simulink library "nonlinlib_config"  (R2013a)
settings: Solver=VariableStepDiscrete  StartTime=0.0  StopTime=10.0  RelTol=1e-3
undefined symbols (not defined in the file or in its folder): Nonlinearity, Tanh
libraries: nonlinlib x1
settings Model: Creator=bbhattac  LastModifiedBy=bbhattac

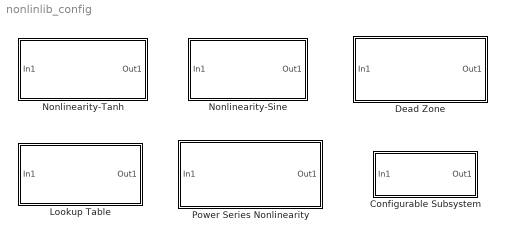
== system nonlinlib_config ==
  Configurable Subsystem : Subsystem  BlockChoice=Nonlinearity-Tanh
      settings: TemplateBlock=self  MemberBlocks=Dead Zone,Lookup Table,Nonlinearity-Sine,Nonlinearity-Tanh,Power Series Nonlinearity
  Dead Zone : Subsystem  mask{range=0.01}
      mask prompts: range "Dead zone half-width"
      mask Display: disp('dead zone');
  Lookup Table : Subsystem
      mask Display: disp('Lookup Table');
  Nonlinearity-Sine : Subsystem  mask{nonlingain=0.2}
      mask prompts: nonlingain "Nonlinear gain"
      mask Display: disp('sin');
  Nonlinearity-Tanh : Subsystem  mask{nonlingain=0.2}
      mask prompts: nonlingain "Nonlinear gain"
      mask Display: disp('tanh');
  Power Series Nonlinearity : Subsystem  mask(Power Series Nonlinearity){nonlingain=1e-05, mu=1e-05}
      mask prompts: nonlingain "Nonlinear factor"; mu "Asymmetry factor"
      mask help: Models the integral nonlinearity of an ADC using 1st order power series.
      mask Help:
      | This block models the integral nonlinearity of an A/D converter using a 1st order power series.
      | Typical values for a high resolution (16 bits or higher) ADC are:
      |   Nonlinear factor = 1.0e-05;
      |   Asymmetry factor = 1.0e-05;
      | 
      | Ref: "Analog-to-Digital Conversion and Harmonic Noises Due to the Integral Nonlinearity," Kiseon Kim, IEEE Trans. Inst. and Meas. Vol. 43, No. 2, pp. 151-156.
      mask Display: disp('Power Series\n Nonlinearity');

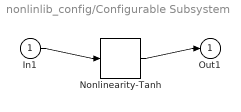
== system nonlinlib_config/Configurable Subsystem ==
  In1 : Inport
  Nonlinearity-Tanh : nonlinlib/Nonlinearity-Tanh  nonlingain=0.2
  Out1 : Outport
  wires:
  In1/1 -> Nonlinearity-Tanh/1
  Nonlinearity-Tanh/1 -> Out1/1

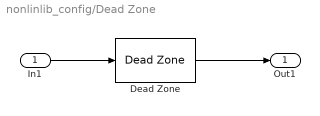
== system nonlinlib_config/Dead Zone ==
  In1 : Inport
  Dead Zone : DeadZone  LowerValue=-range  UpperValue=range  SaturateOnIntegerOverflow=on
  Out1 : Outport
  wires:
  In1/1 -> Dead Zone/1
  Dead Zone/1 -> Out1/1

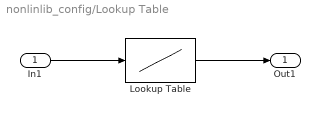
== system nonlinlib_config/Lookup Table ==
  In1 : Inport
  Lookup Table : Lookup  InputValues=[-1, -0.5, 0, 0.5, 1]  Table=[-1, -0.7, 0, 0.7, 1]  LookUpMeth=Interpolation-Use End Values
  Out1 : Outport
  wires:
  Lookup Table/1 -> Out1/1
  In1/1 -> Lookup Table/1

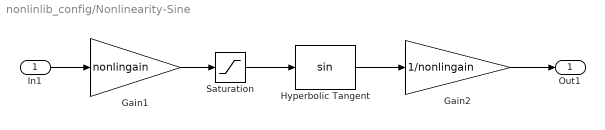
== system nonlinlib_config/Nonlinearity-Sine ==
  In1 : Inport
  Gain1 : Gain  Gain=nonlingain  SaturateOnIntegerOverflow=on  OutDataTypeStr=Inherit: Same as input  ParamDataTypeStr=Inherit: Same as input
  Gain2 : Gain  Gain=1/nonlingain  SaturateOnIntegerOverflow=on  OutDataTypeStr=Inherit: Same as input  ParamDataTypeStr=Inherit: Same as input
  Hyperbolic Tangent : Trigonometry
  Saturation : Saturate  UpperLimit=pi/2  LowerLimit=-pi/2
  Out1 : Outport
  wires:
  Hyperbolic Tangent/1 -> Gain2/1
  Gain1/1 -> Saturation/1
  In1/1 -> Gain1/1
  Gain2/1 -> Out1/1
  Saturation/1 -> Hyperbolic Tangent/1

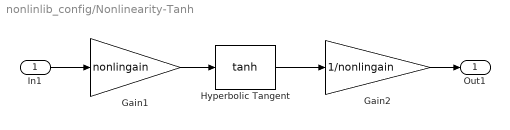
== system nonlinlib_config/Nonlinearity-Tanh ==
  In1 : Inport
  Gain1 : Gain  Gain=nonlingain  SaturateOnIntegerOverflow=on  OutDataTypeStr=Inherit: Same as input  ParamDataTypeStr=Inherit: Same as input
  Gain2 : Gain  Gain=1/nonlingain  SaturateOnIntegerOverflow=on  OutDataTypeStr=Inherit: Same as input  ParamDataTypeStr=Inherit: Same as input
  Hyperbolic Tangent : Trigonometry  Operator=tanh
  Out1 : Outport
  wires:
  Hyperbolic Tangent/1 -> Gain2/1
  Gain1/1 -> Hyperbolic Tangent/1
  In1/1 -> Gain1/1
  Gain2/1 -> Out1/1

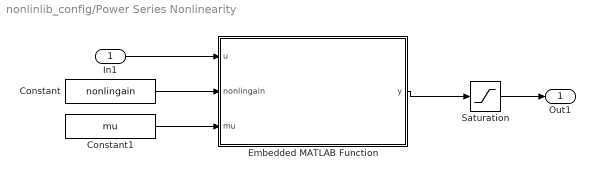
== system nonlinlib_config/Power Series Nonlinearity ==
  In1 : Inport
  Constant : Constant  Value=nonlingain  VectorParams1D=off
  Constant1 : Constant  Value=mu  VectorParams1D=off
  Embedded MATLAB Function : MATLAB Function  TreatAsAtomicUnit=on
  Saturation : Saturate  UpperLimit=1.0  LowerLimit=-1.0
  Out1 : Outport
  wires:
  Constant1/1 -> Embedded MATLAB Function/3(mu)
  Constant/1 -> Embedded MATLAB Function/2(nonlingain)
  Saturation/1 -> Out1/1
  In1/1 -> Embedded MATLAB Function/1(u)
  Embedded MATLAB Function/1(y) -> Saturation/1

== matlab function nonlinlib_config/Power Series Nonlinearity/Embedded MATLAB Function ==
  data: u input; y output; nonlingain input; mu input
function y = ADC_INL(u,nonlingain,mu)
%#eml

if u==0
    y = 0;
elseif u>0
    y = u^(1-nonlingain) + mu*(u^2);
else
    y = -(-u)^(1-nonlingain) + mu*(u^2);
end
